simulink model "Full SWIPT MODEL"  (R2024b)
settings: Solver=VariableStepAuto  StartTime=0.0  StopTime=10  RelTol=1e-3
libraries: commdigbbndpm3 x2, commchan3 x1, commrandsrc3 x1
settings Model: Creator=mpfar  LastModifiedBy=mpfar

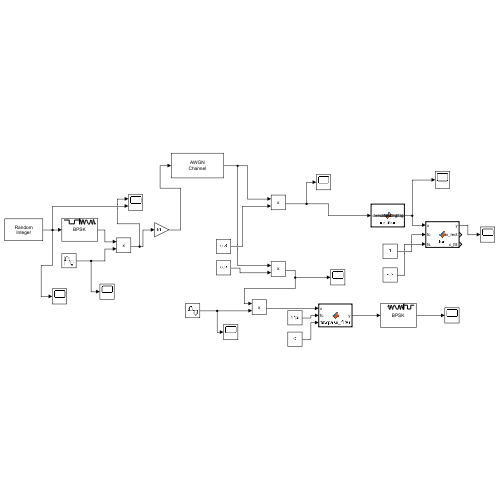
[thumbnail: Simulink's stored preview of the top-level diagram]
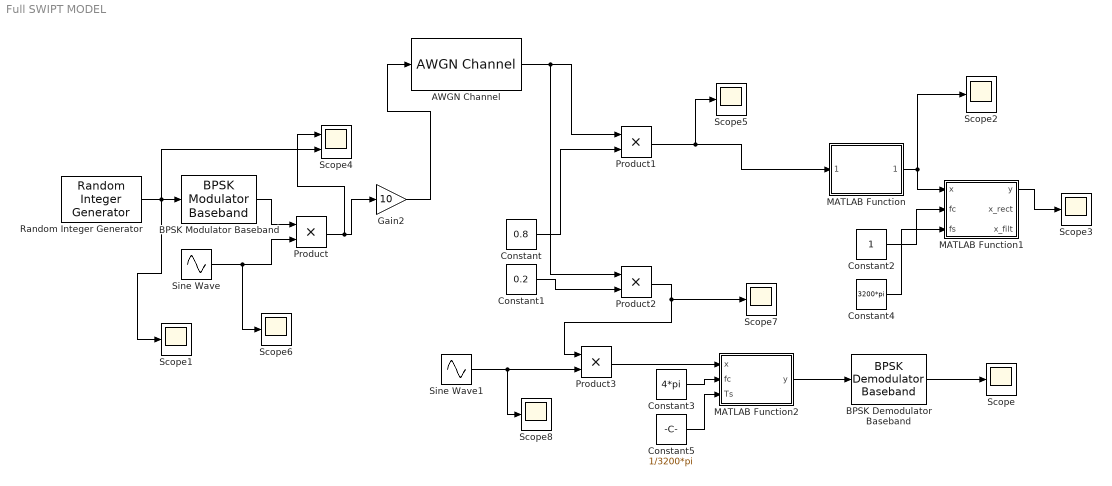
== system Full SWIPT MODEL ==
  AWGN Channel : commchan3/AWGN Channel  LegacyMode=off  NoiseMethod="Signal to noise ratio  (Eb/No)"  noiseMode="Signal to noise ratio  (SNR)"  EbNo=10  EsNo=10  SNR=10  BitsPerSymbol=2  SignalPower=1  SamplesPerSymbol=1  SymbolPeriod=1  VarianceSource=Parameter  Variance=1  RandomStream=Global stream  Seed=67  SimulateUsing=Code generation
  BPSK Demodulator Baseband : commdigbbndpm3/BPSK Demodulator Baseband  DecType=Hard decision  VarSource=Dialog  Variance=1  Ph=0  outDtype=Inherit via internal rule  derotateFactorWordLen=16  derotateFactorDataTypeStr=Inherit: Same word length as input  derotateFactorLastDataTypeStr=Inherit: Same word length as input
      settings: LibrarySourceBlock=|
      | commhdldigbbndpm/BPSK
      | Demodulator
      | Baseband
  BPSK Modulator Baseband : commdigbbndpm3/BPSK Modulator Baseband  Ph=0  outDtype=double  outWordLen=16  outUDDataType=sfix(16)  outFracLenMode=Best precision  outFracLen=15  outDataTypeStr=double  outLastDataTypeStr=double
      settings: LibrarySourceBlock=|
      | commhdldigbbndpm/BPSK
      | Modulator
      | Baseband
  Constant : Constant  Value=0.8
  Constant1 : Constant  Value=0.2
  Constant2 : Constant
  Constant3 : Constant  Value=4*pi
  Constant4 : Constant  Value=3200*pi
  Constant5 : Constant  Value=1/3200*pi
  Gain2 : Gain  Gain=10
  MATLAB Function : MATLAB Function  TreatAsAtomicUnit=on
  MATLAB Function1 : MATLAB Function  TreatAsAtomicUnit=on
  MATLAB Function2 : MATLAB Function  TreatAsAtomicUnit=on
  Product{,1..3} (4 alike) : Product
  Random Integer Generator : commrandsrc3/Random Integer Generator  SetSize=2  SeedSource=Auto  Seed=0  SampleTime=1  SamplesPerFrame=1  OutputDataType=double  SimulateUsing=Interpreted execution
  Scope{,1..3,5..8} (8 alike) : Scope
  Scope4 : Scope  NumInputPorts=2
  Sine Wave : Sin  Frequency=4*pi  SampleTime=1/3200*pi
  Sine Wave1 : Sin  Frequency=4*pi  SampleTime=1/3200*pi
  wires:
  Random Integer Generator/1 -> Scope4/2, Scope1/1, BPSK Modulator Baseband/1
  BPSK Modulator Baseband/1 -> Product/1
  Sine Wave/1 -> Scope6/1, Product/2
  Product/1 -> Scope4/1, Gain2/1
  Constant/1 -> Product1/2
  Constant1/1 -> Product2/2
  Sine Wave1/1 -> Scope8/1, Product3/2
  Product2/1 -> Product3/1, Scope7/1
  Product3/1 -> MATLAB Function2/1(x)
  Constant3/1 -> MATLAB Function2/2(fc)
  Constant5/1 -> MATLAB Function2/3(Ts)
  MATLAB Function2/1(y) -> BPSK Demodulator Baseband/1
  BPSK Demodulator Baseband/1 -> Scope/1
  MATLAB Function/1(rectifiedSignal) -> Scope2/1, MATLAB Function1/1(x)
  Constant2/1 -> MATLAB Function1/2(fc)
  MATLAB Function1/1(y) -> Scope3/1
  Product1/1 -> Scope5/1, MATLAB Function/1(demodulatedSignal)
  Constant4/1 -> MATLAB Function1/3(fs)
  Gain2/1 -> AWGN Channel/1
  AWGN Channel/1 -> Product2/1, Product1/1

== matlab function Full SWIPT MODEL/MATLAB Function1 ==
  data: x input; y output; fc input; fs input; x_rect output; x_filt output
function [y, x_rect, x_filt] = fcn(x, fc, fs)
    persistent b a zi
    if isempty(b)
        % Design a 2nd order Butterworth filter
        [b, a] = butter(2, fc/(fs/2), 'low');
        zi = zeros(max(length(b),length(a))-1, 1);
    end
    
    % Apply rectification
    x_rect = abs(x);
    
    % Apply the Butterworth filter
    [x_filt, zi] = filter(b, a, x_rect, zi);
    
    % Simple moving average
    persistent buffer buffer_index
    if isempty(buffer)
        buffer = zeros(100, 1);  % Adjust buffer size as needed
        buffer_index = 1;
    end
    buffer(buffer_index) = x_filt;
    buffer_index = mod(buffer_index, length(buffer)) + 1;
    y = mean(buffer);
end

== matlab function Full SWIPT MODEL/MATLAB Function ==
  data: demodulatedSignal input; rectifiedSignal output
function rectifiedSignal = rectifier(demodulatedSignal)
    % Rectify the input signal
    rectifiedSignal = abs(demodulatedSignal); % Full-wave rectification
end

== matlab function Full SWIPT MODEL/MATLAB Function2 ==
  data: x input; y output; fc input; Ts input
function y = lowpass_filter(x, fc, Ts)
    % Low-pass filter for complex input signals after downconversion
    % x: Complex input signal (from downconversion)
    % fc: Cutoff frequency of the low-pass filter (Hz)
    % Ts: Sample time (seconds)

    % Declare the output as complex to handle complex input
    y = complex(0);

    % Persistent variable to store the previous output (y[n-1])
    persistent prev_y;
    
    % Initialize prev_y to 0 if this is the first run
    if isempty(prev_y)
        prev_y = complex(0);  % Initialize as complex zero
    end
    
    % Calculate the filter coefficient (alpha) based on the cutoff frequency and sample time
    alpha = 2 * pi * fc * Ts / (2 * pi * fc * Ts + 1);
    
    % Apply the low-pass filter equation: y[n] = alpha * x[n] + (1 - alpha) * y[n-1]
    y = alpha * x + (1 - alpha) * prev_y;
    
    % Store the current output for use in the next iteration (y[n-1] = y[n])
    prev_y = y;
end
